simulink model "may9js"  (R2015a)
settings: Solver=ode4  StartTime=0.0  StopTime=inf  FixedStep=BKIN_STEP_TIME  RelTol=1e-3
StartFcn:
  |  warndlg('Dexterit-E models cannot run under simulation. Please compile your model and run it from within Dexterit-E.');set_param(bdroot,'SimulationCommand','stop')
model workspace (MAT data in the model file):
  BARRIER_ROW = 5
  BKIN_KINEMATIC_FRAME_SIZE = 400
  BKIN_STEP_TIME = 0.00025
  CIRCLE_ROW = 2
  CIRCLE_STROKE = 10
  CIRCLE_STROKE_W = 11
  E_BARRIER_HIT = 6
  E_COLLISION_HIT = 7
  E_ENTER_PRESHOT_AREA = 2
  E_ENTER_START_AREA = 12
  E_EXIT = 13
  E_EXIT_PRESHOT_AREA = 10
  E_GOAL_HIT = 8
  E_GOAL_REACHED = 5
  E_NO_EVENT = 0
  E_PRESHOT_ROW = 4
  E_TARGET_OUT_OF_BOUNDS = 9
  E_TRIAL_BEGIN = 1
  E_TRIAL_ENDED = 3
  FIRST_STATE_FILL = 9
  FORCE_MULTIPLIER = 1
  F_BUMP = 1
  GOAL_ROW = 8
  GOAL_TIME = 15
  HEIGHT = 6
  INVISIBLE_FILL = 15
  LOAD_ROW = 4
  MASS_BARRIER = 6
  MASS_CIRCLE = 2
  MASS_RECT = 3
  NEW_FLOAT = 10
  NEW_ROW = 9
  NEW_TEXTSIZE = 11
  PERT_DUR = 5
  PERT_RAMP = 4
  PRESHOT_ROW = 7
  RADIUS_LOG = 4
  RADIUS_VIS = 5
  RECT_FILL = 12
  RECT_ROW = 3
  RECT_STROKE = 13
  RECT_STROKE_W = 14
  ROTATION = 7
  SECONDS = 1
  SECOND_STATE_FILL = 8
  SHOT_READY_TIME = 13
  SHOT_SET_TIME = 14
  START_HOLD_TIME = 12
  START_ROW = 6
  TRIAL_FAILURE = 11
  WIDTH = 3
  col_x = 1
  col_y = 2
undefined symbols (not defined in the file): slselsubs
libraries: Video x7, General x3, KINARM_loads x2, KINARM_EP_loads x1, KINARM_general x1, simulink x1, slrtlib x1
(part 1 of 4)
settings Model: ModifiedComment=chris -- Wed Feb 16 09:18:30 2005 -- Version 1.1384  ModifiedHistory=Feb 16/05 - Add error repeat, add offset ramp  ExtModeArmWhenConnect=off  ExtModeLogAll=off  Creator=Chris Grebeldinger  LastModifiedBy=User
settings SolverCC: AutoInsertRateTranBlk=on
settings DataIOCC: LimitDataPoints=off  SignalLoggingSaveFormat=ModelDataLogs  SaveOutput=off  SaveTime=off  SignalLoggingName=sigsOut
settings OptimizationCC: BlockReduction=off  BooleanDataType=off  OptimizeBlockIOStorage=off  BufferReuse=off  GlobalBufferReuse=off  ExpressionFolding=off  ExpressionDepthLimit=2147483647  LocalBlockOutputs=off  InitFltsAndDblsToZero=on
settings DebuggingCC: SaveWithParameterizedLinksMsg=none  UnderspecifiedInitializationDetection=Classic  MergeDetectMultiDrivingBlocksExec=none  SignalResolutionControl=TryResolveAllWithWarning  MultiTaskDSMMsg=warning  FcnCallInpInsideContextMsg=EnableAllAsWarning  BusObjectLabelMismatch=none  StateNameClashWarn=warning  StrictBusMsg=ErrorOnBusTreatedAsVector
settings HardwareCC: ProdIntDivRoundTo=Zero  ProdEndianess=LittleEndian  ProdLongLongMode=on  ProdHWDeviceType=Generic->32-bit x86 compatible  TargetHWDeviceType=32-bit Generic
settings SFSimCC: SimParseCustomCode=off
settings RTWCC: Description=Simulink Real-Time  SystemTargetFile=slrt.tlc  TemplateMakefile=slrt_default_tmf  CodeExecutionProfiling=on  RTWCompilerOptimization=on
settings CodeAppCC: MaxIdLength=63
settings SimulinkRealTimeCC: TargetFcnLib=ansi_tfl_tmw.mat  GeneratePreprocessorConditionals=Disable all

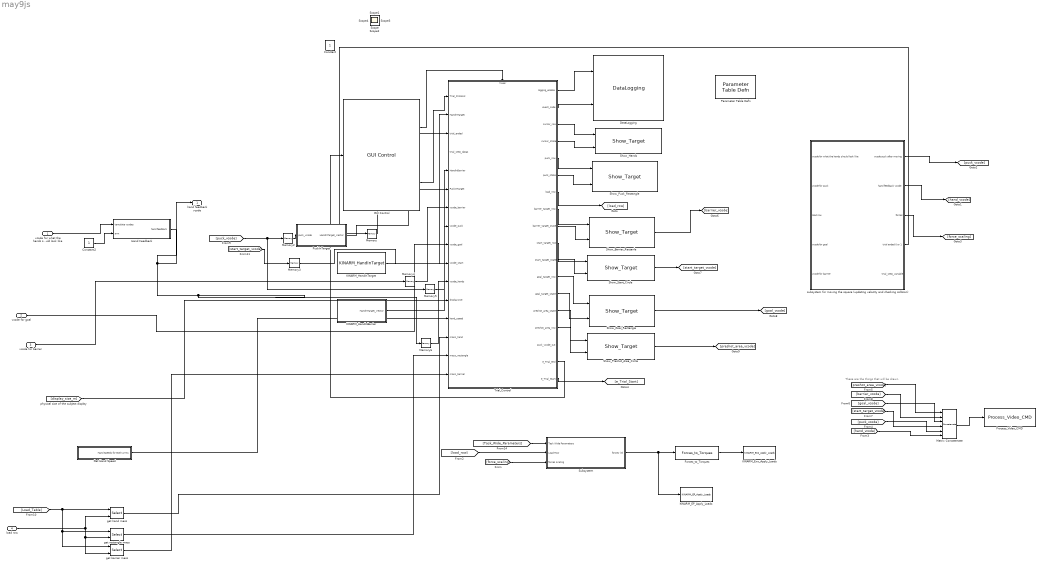
== system may9js ==
  note: These are the things that will be drawn
  vcode for what the hands should look like : Inport  PortDimensions=[1 70]
  vcode for goal : Inport  Port=2  PortDimensions=[1 70]
  vcode for barrier : Inport  Port=3  PortDimensions=[1 70]
  load row : Inport  Port=4
  Constant2 : Constant
  DataLogging : General/DataLogging  log_event_codes=on  log_analog_inputs=off  show_time_remaining=off  ecat_include=on
  Forces_to_Torques : KINARM_loads/Forces_to_Torques
  GUI Control : General/GUI Control  task_version=1.0  show_repeat_trial_flag=off  use_custom_tp=off  target_type_str=Circle  Target_Type=1  XYcols=[1 2]  Vcols=3  Lcols=4  indices_padding=[0 0 0 0;0 0 0 0]  target_table_rows=64  load_table_rows=20  tp_table_rows=100
  Get Hand Speed : Subsystem
  Hand Feedback : Subsystem
  KINARM_EP_Apply_Loads : KINARM_EP_loads/KINARM_EP_Apply_Loads  up_duration=1500  down_duration=1500  max_force=20
  KINARM_Exo_Apply_Loads : KINARM_loads/KINARM_Exo_Apply_Loads  up_duration=1500  down_duration=1500  max_torque=5  limit_motors=off
  KINARM_HandInBarrier : Subsystem  AncestorBlock=KINARM_general/KINARM_HandInTarget  mask(KINARM_HandInTarget){use_dominant_hand=on, target_type=Rectangle, num_states=1, attribcol1=[WIDTH HEIGHT ROTATION], attribcol2=[0 0 0], attribcol3=[0 0 0], attribcol4=[0 0 0], attribcol5=[0 0 0]}
      mask prompts: use_dominant_hand "Use "arm to be assessed"?"; target_type "Type of Target"; num_states "Number of Target States"; attribcol1 "State 1 Target Table Column(s)"; attribcol2 "State 2 Target Table Column(s)"; attribcol3 "State 3 Target Table Column(s)"; attribcol4 "State 4 Target Table Column(s)"; attribcol5 "State 5 Target Table Column(s)"
      mask help: This block returns a vector or array corresponding to the Target_Table rows indicating whether the specified hand is in (=1) or out (=0) of each of the targets.
      mask init:
      | block_path = gcb;  % store block path, as gcb may change with block operations
      | 
      | %%% Get the model's workspace, because it is required to evaluate constants from the Parameter Table Def'n block
      | modelName=bdroot(block_path);
      | modelWorkspace = get_param(modelName, 'ModelWorkspace');
      | 
      | %%% Handle background colours if link status changes.  
      | checkBackgroundColour(block_path, 'KINARM_general');
      | 
      | %%% create the names of the input and output ports to display on the mask
      | % Select only the desired states for output. The output port is also renamed to reflect 
      | % whether the output is a vector (in the case of a single state) or an array (of vectors, 
      | % one for each of multiple states).
      | 
      | numStates = str2double( get_param(block_path, 'num_states') );
      | 
      | if numStates == 1
      | 	set_param([block_path '/Selected States'], 'Value', '[1]');
      | 	outputname = 'HandInTarget_Vector';
      | elseif numStates == 2
      | 	set_param([block_path '/Selected States'], 'Value', '[1,2]');
      | 	outputname = 'HandInTarget_Array';
      | elseif numStates == 3
      | 	set_param([block_path '/Selected States'], 'Value', '[1,2,3]');
      | 	outputname = 'HandInTarget_Array';
      | elseif numStates == 4
      | 	set_param([block_path '/Selected States'], 'Value', '[1,2,3,4]');
      | 	outputname = 'HandInTarget_Array';
      | else
      | 	set_param([block_path '/Selected States'], 'Value', '[1,2,3,4,5]');
      | 	outputname = 'HandInTarget_Array';
      | end
      | output_block=char(find_system(gcb,'LookUnderMasks','all','FollowLinks','on','SearchDepth',1,'BlockType','Outport'));
      | set_param(output_block, 'Name', outputname);
      | 
      | 
      | %%%%%%%%%%%%%%%%%%%%%%%%%%%%%%%%%%%%%%%%%%%%%%%%%%%%%%%%%%%%%
      | %%% Check and format the input strings for the vectors of column entires
      | targetTypeStr=get_param(block_path, 'target_type');
      | 
      | switch targetTypeStr(1:3)
      | 	case 'Cir',		numCol = 1;
      | 	case 'Ell',		numCol = 3;
      |     case 'Rec',		numCol = 3;
      |     case 'Lin',		numCol = 3;
      |     case 'Tri',		numCol = 4;
      | 	otherwise,		numCol = 1;
      | end
      | 
      | for ii = 1:numStates
      | 	variableName = ['attribcol' num2str(ii)];
      | 	attribcoltext = get_param(block_path, variableName);
      | 	attribcoltext = checkUserInputVectorLength(attribcoltext, numCol);
      | 	set_param(block_path, variableName, attribcoltext);
      | end
      | 
      | for ii = 1+numStates:5
      | 	variableName = ['attribcol' num2str(ii)];
      |     if numCol == 1
      |         outstr = '[0]';
      |     else
      |         outstr = mat2str(zeros(1, numCol));
      |     end
      |     set_param(block_path, variableName, outstr);
      | end
      | 
      | %%%%%%%%%%%%%%%%%%%%%%%%%%%%%%%%%%%%%%%%%%%%%%%%%%%%%%%%%%%%%
      | %%% Create the text to show on the mask
      | numStates = str2num(get_param(block_path, 'num_states'));
      | columntext='(columns: ';
      | 
      | for ii = 1:numStates
      | 	variableName = ['attribcol' num2str(ii)];
      | 	attribcolString = get_param(block_path, variableName);
      | 	if isempty(modelWorkspace)
      | 		% if the block is part of a library, then modelWorkspace will be empty and the other code to evaluate attribcolStringEval will fail
      | 		attribcolStringEval = '3';
      | 	else
      | 		[attribcolValue, errorMessage] = BKINevalin(modelWorkspace, attribcolString);
      | 		attribcolStringEval = mat2str( attribcolValue );
      | 	end
      | 	if ii > 1
      | 		columntext = [columntext, '; ', attribcolStringEval];
      | 	else
      | 		columntext = [columntext, attribcolStringEval];
      | 	end
      | end
      | 
      | % Add formatting spaces so that the mask looks nice
      | columntext=strvcat([columntext ')'],' ', ' ');
      mask Help:
      | Used to determine if the hand (fingertip) is in any of the targets in the Target_Table.
      | <P>
      | <B><I>Use of this block requires that the DataLogging block (General library) be set to log KINARM data.</I></B>
      | 
      | <H2>Library </H2>
      | KINARM general
      | 
      | <H2>Description </H2>
      | This block returns a vector or array corresponding to the Target_Table rows indicating whether the specified hand (i.e. fingertip) is in or out of each of the targets.  Each element in the output vector or output array will be either a 0 (hand not in target) or a 1 (hand in target).
      | <P>
      | A vector is returned if only one target state is specified in each target row (see Parameters and Dialog Box), with each index of the vector corresponding to a row in the target table.  An array is returned if more than one target state is specified in a target row, with each row of the array corresponding to a target row and each column corresponding to the nth target state specified in each target row.
      | <P>
      | The output vector or array is typically used by a stateflow chart to affect behavior of the system.  Because this block returns hand-in-target information for all targets in the target table, multiple targets can be monitored at once (i.e. the Stateflow chart could have certain transitions that occur if the hand is in one target and other transitions if it is in a different target).  Likewise, because this block returns hand-in-target information for multiple states of a single target, those multiple states can be monitored simultaneously.
      | <P>
      | Because the KINARM_HandInTarget block returns information for only one hand, two copies of this block are required if information for both hands is desired.
      | <P>
      | 
      | <H2>Parameters and Dialog Box</H2>
      | <B>Use "arm to be assessed"?:</B> this checkbox determines which hand is used by this block. In Dexterit-E the operator selects the "arm to be assessed" using radio buttons.
      | When this box is checked the output of this block is derived from the hand information corresponding to the arm selection made by the operator in Dexterit-E.
      | When this box is unchecked the output of this block is derived from the contralateral arm.
      | (Note: to obtain information about both hands, then 2 separate copies of this block are required - one for each hand.)
      | <P>
      | <B>Type of Target:</B> Enter the type of target specified in the target table:
      | <P>
      | <B>Number of Target States:</B> Enter the number of target states specified in each target row.  Up to four target states are allowed per target row.
      | <P>
      | <B>State <n> Target Table Columns:</B> Enter the columns in the Target Table that specify the relevant target attributes.  Do this for each target state.
      | For a circle, enter the columns corresponding to logical radius (e.g. 4)
      | <BR>For an ellipse, enter the columns corresponding to major radius, minor radius, rotation angle (e.g. [4, 5, 6]).
      | <BR>For a rectangle, enter the columns corresponding to length, height, and rotation angle (e.g. [4, 5, 6]).
      | <BR>For a line, enter the columns corresponding to stroke width, endpoint in x, and endpoint in y (e.g. [3, 4, 5]).
      | <BR>For a triangle, enter the columns corresponding to length, height, peak offset, and rotation angle (e.g. [4, 5, 6, 7]).
      | 
      | <H2>Examples</H2>
      | <B>Example 1.</B>  Suppose a target row will be used to define 1 state for a circle type target and the radius of the visual target is the same radius to be used for determination of hand-in-target.  The related Target Table column is: column 6 = radius.  For this example, "State 1 Target Table Columns" would equal [6].
      | <P>
      | 
      | <B>Example 2.</B>  Suppose a target row will be used to define 1 state for a circle type target, but the radius of the visual target will be different than the radius to be used for determination of hand-in-target.  This option allows independent control over the size of the visual target versus the accuracy needed to be considered "in the target".  The related Target Table columns are: column 6 = radius1 (i.e. radius to target to be drawn); column 7 = radius2 (i.e. radius to be used for hand-in-target) .  For this example, "State 1 Target Table Columns" would equal [7].
      | <P>
      | <B>Example 3.</B>  Suppose a target row will be used to define 2 states for a circle type target, where the radius of the visual target will be a constant, but depending on the state of the system, one of 2 other and different radii will be used for determination of hand-in-target.  The related Target Table columns are: column 6 = radius1 (i.e. radius to target to be drawn); column 7 = radius2 (i.e. radius to be used for hand-in-target for state 1); column 8 = radius3 (i.e. radius to be used for hand-in-target for state 2).  For this example, "State 1 Target Table Columns" would equal [7], while "State 2 Target Table Columns" would equal [8].
      | <P>
      | 
      | <H2>Related Blocks </H2>
      | DataLogging
      mask TypeOptions target_type: Circle | Ellipse | Rectangle | Line | Triangle
      mask Callback target_type:
      | %%%%
      | % Because of bugs iN R2007, R2010a and R2013a (which have been reported to Mathworks), the following code
      | % is required here because in the Initialization Section it will ONLY correctly update those Mask Parameters that are hidden
      | % when the OK button is clicked (NOTE: the initialization code will correctly update all Mask Parameters when the Apply button
      | % is clicked, the bug is that it should also update everything when the OK button is clicked in the absence of an Apply click)
      | %
      | % Adding a set_param call which updates one of the mask parameters will call the initialization code to run, which "avoids"
      | % this bug. This code should be removed once Mathworks has fixed this bug.
      | 
      | temp = get_param(gcb, 'target_type');
      | set_param(gcb, 'target_type', temp);
      mask TypeOptions num_states: 1 | 2 | 3 | 4 | 5
      mask Callback num_states:
      | num_states = str2num(get_param(gcb, 'num_states'));
      | vis = get_param(gcb, 'MaskVisibilities');
      | 
      | % Select only the desired states for output. The output port is also renamed to reflect
      | % whether the output is a vector (in the case of a single state) or an array (of vectors,
      | % one for each of multiple states).
      | output_block=char(find_system(gcb, 'LookUnderMasks', 'all', 'FollowLinks', 'on', 'SearchDepth', 1, 'BlockType', 'Outport'));
      | 
      | if num_states == 1
      | % % % 	set_param([gcb '/Selected States'], 'Value', '[1]');
      | % % % 	set_param(output_block, 'Name', 'HandInTarget_Vector');
      | 	vis{5} = 'off';
      | 	vis{6} = 'off';
      | 	vis{7} = 'off';
      | 	vis{8} = 'off';
      | elseif num_states == 2
      | % % % 	set_param([gcb '/Selected States'], 'Value', '[1,2]');
      | % % % 	set_param(output_block, 'Name', 'HandInTarget_Array');
      | 	vis{5} = 'on';
      | 	vis{6} = 'off';
      | 	vis{7} = 'off';
      | 	vis{8} = 'off';
      | elseif num_states == 3
      | % % % 	set_param([gcb '/Selected States'], 'Value', '[1,2,3]');
      | % % % 	set_param(output_block, 'Name','HandInTarget_Array');
      | 	vis{5} = 'on';
      | 	vis{6} = 'on';
      | 	vis{7} = 'off';
      | 	vis{8} = 'off';
      | elseif num_states == 4
      | % % % 	set_param([gcb '/Selected States'], 'Value', '[1,2,3,4]');
      | % % % 	set_param(output_block, 'Name','HandInTarget_Array');
      | 	vis{5} = 'on';
      | 	vis{6} = 'on';
      | 	vis{7} = 'on';
      | 	vis{8} = 'off';
      | else
      | % % % 	set_param([gcb '/Selected States'], 'Value', '[1,2,3,4,5]');
      | % % % 	set_param(output_block, 'Name', 'HandInTarget_Array');
      | 	vis{5} = 'on';
      | 	vis{6} = 'on';
      | 	vis{7} = 'on';
      | 	vis{8} = 'on';
      | end
      | set_param(gcb, 'MaskVisibilities', vis);
      mask Display:
      | disp(columntext);
      | port_label('output',1,outputname);
  KINARM_HandInTarget : KINARM_general/KINARM_HandInTarget  use_dominant_hand=on  target_type=Circle  num_states=1  attribcol1=[RADIUS_LOG]  attribcol2=[0]  attribcol3=[0]  attribcol4=[0]  attribcol5=[0]
  Matrix Concatenate : Concatenate  NumInputs=6  Mode=Multidimensional array
  Memory{,2..6} (6 alike) : Memory
  Parameter Table Defn : General/Parameter Table Defn  ShowInLibBrowser=0
  Process_Video_CMD : Video/Process_Video_CMD  video_delay=0
  PuckInTarget : Subsystem  AncestorBlock=KINARM_general/KINARM_HandInTarget  mask(KINARM_HandInTarget){use_dominant_hand=on, target_type=Rectangle, num_states=1, attribcol1=[WIDTH HEIGHT ROTATION], attribcol2=[0 0 0], attribcol3=[0 0 0], attribcol4=[0 0 0], attribcol5=[0 0 0]}
      mask prompts: use_dominant_hand "Use "arm to be assessed"?"; target_type "Type of Target"; num_states "Number of Target States"; attribcol1 "State 1 Target Table Column(s)"; attribcol2 "State 2 Target Table Column(s)"; attribcol3 "State 3 Target Table Column(s)"; attribcol4 "State 4 Target Table Column(s)"; attribcol5 "State 5 Target Table Column(s)"
      mask help: This block returns a vector or array corresponding to the Target_Table rows indicating whether the specified hand is in (=1) or out (=0) of each of the targets.
      mask init: same as may9js/KINARM_HandInBarrier
      mask Help:
      | Used to determine if the hand (fingertip) is in any of the targets in the Target_Table.
      | <P>
      | <B><I>Use of this block requires that the DataLogging block (General library) be set to log KINARM data.</I></B>
      | 
      | <H2>Library </H2>
      | KINARM general
      | 
      | <H2>Description </H2>
      | This block returns a vector or array corresponding to the Target_Table rows indicating whether the specified hand (i.e. fingertip) is in or out of each of the targets.  Each element in the output vector or output array will be either a 0 (hand not in target) or a 1 (hand in target).
      | <P>
      | A vector is returned if only one target state is specified in each target row (see Parameters and Dialog Box), with each index of the vector corresponding to a row in the target table.  An array is returned if more than one target state is specified in a target row, with each row of the array corresponding to a target row and each column corresponding to the nth target state specified in each target row.
      | <P>
      | The output vector or array is typically used by a stateflow chart to affect behavior of the system.  Because this block returns hand-in-target information for all targets in the target table, multiple targets can be monitored at once (i.e. the Stateflow chart could have certain transitions that occur if the hand is in one target and other transitions if it is in a different target).  Likewise, because this block returns hand-in-target information for multiple states of a single target, those multiple states can be monitored simultaneously.
      | <P>
      | Because the KINARM_HandInTarget block returns information for only one hand, two copies of this block are required if information for both hands is desired.
      | <P>
      | 
      | <H2>Parameters and Dialog Box</H2>
      | <B>Use "arm to be assessed"?:</B> this checkbox determines which hand is used by this block. In Dexterit-E the operator selects the "arm to be assessed" using radio buttons.
      | When this box is checked the output of this block is derived from the hand information corresponding to the arm selection made by the operator in Dexterit-E.
      | When this box is unchecked the output of this block is derived from the contralateral arm.
      | (Note: to obtain information about both hands, then 2 separate copies of this block are required - one for each hand.)
      | <P>
      | <B>Type of Target:</B> Enter the type of target specified in the target table:
      | <P>
      | <B>Number of Target States:</B> Enter the number of target states specified in each target row.  Up to four target states are allowed per target row.
      | <P>
      | <B>State <n> Target Table Columns:</B> Enter the columns in the Target Table that specify the relevant target attributes.  Do this for each target state.
      | For a circle, enter the columns corresponding to logical radius (e.g. 4)
      | <BR>For an ellipse, enter the columns corresponding to major radius, minor radius, rotation angle (e.g. [4, 5, 6]).
      | <BR>For a rectangle, enter the columns corresponding to length, height, and rotation angle (e.g. [4, 5, 6]).
      | <BR>For a line, enter the columns corresponding to stroke width, endpoint in x, and endpoint in y (e.g. [3, 4, 5]).
      | <BR>For a triangle, enter the columns corresponding to length, height, peak offset, and rotation angle (e.g. [4, 5, 6, 7]).
      | 
      | <H2>Examples</H2>
      | <B>Example 1.</B>  Suppose a target row will be used to define 1 state for a circle type target and the radius of the visual target is the same radius to be used for determination of hand-in-target.  The related Target Table column is: column 6 = radius.  For this example, "State 1 Target Table Columns" would equal [6].
      | <P>
      | 
      | <B>Example 2.</B>  Suppose a target row will be used to define 1 state for a circle type target, but the radius of the visual target will be different than the radius to be used for determination of hand-in-target.  This option allows independent control over the size of the visual target versus the accuracy needed to be considered "in the target".  The related Target Table columns are: column 6 = radius1 (i.e. radius to target to be drawn); column 7 = radius2 (i.e. radius to be used for hand-in-target) .  For this example, "State 1 Target Table Columns" would equal [7].
      | <P>
      | <B>Example 3.</B>  Suppose a target row will be used to define 2 states for a circle type target, where the radius of the visual target will be a constant, but depending on the state of the system, one of 2 other and different radii will be used for determination of hand-in-target.  The related Target Table columns are: column 6 = radius1 (i.e. radius to target to be drawn); column 7 = radius2 (i.e. radius to be used for hand-in-target for state 1); column 8 = radius3 (i.e. radius to be used for hand-in-target for state 2).  For this example, "State 1 Target Table Columns" would equal [7], while "State 2 Target Table Columns" would equal [8].
      | <P>
      | 
      | <H2>Related Blocks </H2>
      | DataLogging
      mask TypeOptions target_type: Circle | Ellipse | Rectangle | Line | Triangle
      mask Callback target_type:
      | %%%%
      | % Because of bugs iN R2007, R2010a and R2013a (which have been reported to Mathworks), the following code
      | % is required here because in the Initialization Section it will ONLY correctly update those Mask Parameters that are hidden
      | % when the OK button is clicked (NOTE: the initialization code will correctly update all Mask Parameters when the Apply button
      | % is clicked, the bug is that it should also update everything when the OK button is clicked in the absence of an Apply click)
      | %
      | % Adding a set_param call which updates one of the mask parameters will call the initialization code to run, which "avoids"
      | % this bug. This code should be removed once Mathworks has fixed this bug.
      | 
      | temp = get_param(gcb, 'target_type');
      | set_param(gcb, 'target_type', temp);
      mask TypeOptions num_states: 1 | 2 | 3 | 4 | 5
      mask Callback num_states:
      | num_states = str2num(get_param(gcb, 'num_states'));
      | vis = get_param(gcb, 'MaskVisibilities');
      | 
      | % Select only the desired states for output. The output port is also renamed to reflect
      | % whether the output is a vector (in the case of a single state) or an array (of vectors,
      | % one for each of multiple states).
      | output_block=char(find_system(gcb, 'LookUnderMasks', 'all', 'FollowLinks', 'on', 'SearchDepth', 1, 'BlockType', 'Outport'));
      | 
      | if num_states == 1
      | % % % 	set_param([gcb '/Selected States'], 'Value', '[1]');
      | % % % 	set_param(output_block, 'Name', 'HandInTarget_Vector');
      | 	vis{5} = 'off';
      | 	vis{6} = 'off';
      | 	vis{7} = 'off';
      | 	vis{8} = 'off';
      | elseif num_states == 2
      | % % % 	set_param([gcb '/Selected States'], 'Value', '[1,2]');
      | % % % 	set_param(output_block, 'Name', 'HandInTarget_Array');
      | 	vis{5} = 'on';
      | 	vis{6} = 'off';
      | 	vis{7} = 'off';
      | 	vis{8} = 'off';
      | elseif num_states == 3
      | % % % 	set_param([gcb '/Selected States'], 'Value', '[1,2,3]');
      | % % % 	set_param(output_block, 'Name','HandInTarget_Array');
      | 	vis{5} = 'on';
      | 	vis{6} = 'on';
      | 	vis{7} = 'off';
      | 	vis{8} = 'off';
      | elseif num_states == 4
      | % % % 	set_param([gcb '/Selected States'], 'Value', '[1,2,3,4]');
      | % % % 	set_param(output_block, 'Name','HandInTarget_Array');
      | 	vis{5} = 'on';
      | 	vis{6} = 'on';
      | 	vis{7} = 'on';
      | 	vis{8} = 'off';
      | else
      | % % % 	set_param([gcb '/Selected States'], 'Value', '[1,2,3,4,5]');
      | % % % 	set_param(output_block, 'Name', 'HandInTarget_Array');
      | 	vis{5} = 'on';
      | 	vis{6} = 'on';
      | 	vis{7} = 'on';
      | 	vis{8} = 'on';
      | end
      | set_param(gcb, 'MaskVisibilities', vis);
      mask Display:
      | disp(columntext);
      | port_label('output',1,outputname);
  Show_Barrier_Rectanle : Video/Show_Target  target_type=Rectangle  num_states=2  attribcol1=[FIRST_STATE_FILL RECT_STROKE RECT_STROKE_W WIDTH HEIGHT ROTATION]  attribcol2=[SECOND_STATE_FILL RECT_STROKE RECT_STROKE_W WIDTH HEIGHT ROTATION]  attribcol3=[0 0 0 0 0 0]  attribcol4=[0 0 0 0 0 0]  attribcol5=[0 0 0 0 0 0]  stateindices_padding=[0 0 0 0 0;0 0 0 0 0;0 0 0 0 0;0 0 0 0 0;0 0 0 0 0]  source=dialog  opacity=100  target_display=Both subject and operator displays  num_col=6
  Show_Goal_Rectangle : Video/Show_Target  target_type=Rectangle  num_states=3  attribcol1=[INVISIBLE_FILL RECT_STROKE RECT_STROKE_W WIDTH HEIGHT ROTATION]  attribcol2=[FIRST_STATE_FILL RECT_STROKE RECT_STROKE_W WIDTH HEIGHT ROTATION]  attribcol3=[SECOND_STATE_FILL RECT_STROKE RECT_STROKE_W WIDTH HEIGHT ROTATION]  attribcol4=[0 0 0 0 0 0]  attribcol5=[0 0 0 0 0 0]  stateindices_padding=[0 0 0 0 0;0 0 0 0 0;0 0 0 0 0;0 0 0 0 0;0 0 0 0 0]  source=dialog  opacity=100  target_display=Both subject and operator displays  num_col=6
  Show_Hands : Video/Show_Target  target_type=Circle  num_states=2  attribcol1=[FIRST_STATE_FILL CIRCLE_STROKE CIRCLE_STROKE_W WIDTH]  attribcol2=[SECOND_STATE_FILL CIRCLE_STROKE CIRCLE_STROKE_W WIDTH]  attribcol3=[0 0 0 0]  attribcol4=[0 0 0 0]  attribcol5=[0 0 0 0]  stateindices_padding=[0 0 0 0 0 0 0;0 0 0 0 0 0 0;0 0 0 0 0 0 0;0 0 0 0 0 0 0;0 0 0 0 0 0 0]  source=dialog  opacity=100  target_display=Both subject and operator displays  num_col=4
  Show_Preshot_Area_Circle : Video/Show_Target  target_type=Circle  num_states=3  attribcol1=[INVISIBLE_FILL CIRCLE_STROKE CIRCLE_STROKE_W WIDTH]  attribcol2=[FIRST_STATE_FILL CIRCLE_STROKE CIRCLE_STROKE_W WIDTH]  attribcol3=[SECOND_STATE_FILL CIRCLE_STROKE CIRCLE_STROKE_W WIDTH]  attribcol4=[0 0 0 0]  attribcol5=[0 0 0 0]  stateindices_padding=[0 0 0 0 0 0 0;0 0 0 0 0 0 0;0 0 0 0 0 0 0;0 0 0 0 0 0 0;0 0 0 0 0 0 0]  source=dialog  opacity=100  target_display=Both subject and operator displays  num_col=4
  Show_Puck_Rectangle : Video/Show_Target  target_type=Rectangle  num_states=3  attribcol1=[INVISIBLE_FILL RECT_STROKE RECT_STROKE_W WIDTH HEIGHT ROTATION]  attribcol2=[FIRST_STATE_FILL RECT_STROKE RECT_STROKE_W WIDTH HEIGHT ROTATION]  attribcol3=[SECOND_STATE_FILL RECT_STROKE RECT_STROKE_W WIDTH HEIGHT ROTATION]  attribcol4=[0 0 0 0 0 0]  attribcol5=[0 0 0 0 0 0]  stateindices_padding=[0 0 0 0 0;0 0 0 0 0;0 0 0 0 0;0 0 0 0 0;0 0 0 0 0]  source=dialog  opacity=100  target_display=Both subject and operator displays  num_col=6
  Show_Start_Circle : Video/Show_Target  target_type=Circle  num_states=3  attribcol1=[INVISIBLE_FILL CIRCLE_STROKE CIRCLE_STROKE_W WIDTH]  attribcol2=[FIRST_STATE_FILL CIRCLE_STROKE CIRCLE_STROKE_W WIDTH]  attribcol3=[SECOND_STATE_FILL CIRCLE_STROKE CIRCLE_STROKE_W WIDTH]  attribcol4=[0 0 0 0]  attribcol5=[0 0 0 0]  stateindices_padding=[0 0 0 0 0 0 0;0 0 0 0 0 0 0;0 0 0 0 0 0 0;0 0 0 0 0 0 0;0 0 0 0 0 0 0]  source=dialog  opacity=100  target_display=Both subject and operator displays  num_col=4
  Subsystem : Subsystem
  Trial_Control : Stateflow chart  TreatAsAtomicUnit=on
      settings: PermitHierarchicalResolution=ParametersOnly
  get barrier mass : Selector  NumberOfDimensions=2  IndexOptions=Index vector (port),Index vector (dialog)  Indices=MASS_RECT,MASS_RECT  OutputSizes=1,1
  get hand mass : Selector  NumberOfDimensions=2  IndexOptions=Index vector (port),Index vector (dialog)  Indices=MASS_CIRCLE,MASS_CIRCLE  OutputSizes=1,1
  get rectangle mass : Selector  NumberOfDimensions=2  IndexOptions=Index vector (port),Index vector (dialog)  Indices=MASS_RECT,MASS_RECT  OutputSizes=1,1
  subsystem for moving the square (updating velocity and checking collision) : Subsystem
  hand feedback vcode : Outport
  Constant : Constant  IOType=siggen
  Scope{,1..4} (5 alike) : Scope
      Scope settings: TimeRange=auto  MaxDataPoints=5000  SaveToWorkspace=off  SaveName=ScopeData  YMin=-10.00000  YMax=10.00000  SampleTime=-1
      Scope1 settings: TimeRange=auto  MaxDataPoints=5000  SaveToWorkspace=off  YMin=-10.00000  YMax=10.00000  SampleTime=-1
      Scope2 settings: TimeRange=auto  MaxDataPoints=5000  SaveToWorkspace=off  SaveName=ScopeData2  YMin=-10.00000  YMax=10.00000  SampleTime=-1
      Scope3 settings: TimeRange=auto  MaxDataPoints=5000  SaveToWorkspace=off  SaveName=ScopeData3  YMin=-10.00000  YMax=10.00000  SampleTime=-1
      Scope4 settings: TimeRange=auto  MaxDataPoints=5000  SaveToWorkspace=off  SaveName=ScopeData4  YMin=-10.00000  YMax=10.00000  SampleTime=-1
  wires:
  Trial_Control/3(cursor_row) -> Show_Hands/1
  Trial_Control/5(puck_row) -> Show_Puck_Rectangle/1
  Trial_Control/6(puck_state) -> Show_Puck_Rectangle/2
  Forces_to_Torques/1 -> KINARM_Exo_Apply_Loads/1
  Trial_Control/1(logging_enable) -> DataLogging/1
  Trial_Control/7(load_row) -> [load_row]
  Trial_Control/17(e_Trial_End) -> GUI Control/1
  Trial_Control/4(cursor_state) -> Show_Hands/2
  GUI Control/1 -> Trial_Control/Trigger
  Matrix Concatenate/1 -> Process_Video_CMD/1
  subsystem for moving the square (updating velocity and checking collision)/1(vcode puck after moving) -> [puck_vcode]
  subsystem for moving the square (updating velocity and checking collision)/3(forces) -> [force_scaling]
  subsystem for moving the square (updating velocity and checking collision)/2(hand feedback vcode) -> [hand_vcode]
  Trial_Control/2(event_code) -> DataLogging/2
  Subsystem/1(forces (N)) -> KINARM_EP_Apply_Loads/1, Forces_to_Torques/1
  [Task_Wide_Parameters] -> Subsystem/1(Task Wide Parameters)
  [load_row] -> Subsystem/2(Load Row)
  [force_scaling] -> Subsystem/3(forces scaling)
  Trial_Control/8(barrier_target_row) -> Show_Barrier_Rectanle/1
  Trial_Control/9(barrier_target_state) -> Show_Barrier_Rectanle/2
  Trial_Control/10(start_target_row) -> Show_Start_Circle/1
  Trial_Control/11(start_target_state) -> Show_Start_Circle/2
  Trial_Control/12(goal_target_row) -> Show_Goal_Rectangle/1
  Trial_Control/13(goal_target_state) -> Show_Goal_Rectangle/2
  KINARM_HandInTarget/1 -> Trial_Control/2(HandInTarget)
  GUI Control/2 -> Trial_Control/1(Trial_Protocol)
  subsystem for moving the square (updating velocity and checking collision)/4(trial ended 0 or 1) -> Memory/1
  Memory/1 -> Trial_Control/3(trial_ended)
  Show_Barrier_Rectanle/1 -> [barrier_vcode]
  Show_Start_Circle/1 -> [start_target_vcode]
  Trial_Control/14(preshot_area_state) -> Show_Preshot_Area_Circle/2
  Trial_Control/15(preshot_area_row) -> Show_Preshot_Area_Circle/1
  [hand_vcode] -> Matrix Concatenate/6
  [puck_vcode] -> Matrix Concatenate/5
  [preshot_area_vcode] -> Matrix Concatenate/1
  [barrier_vcode] -> Matrix Concatenate/2
  [goal_vcode] -> Matrix Concatenate/3
  [start_target_vcode] -> Matrix Concatenate/4
  KINARM_HandInBarrier/1(HandInTarget_Vector) -> Trial_Control/5(HandInBarrier)
  [puck_vcode] -> Memory5/1, Memory2/1
  PuckInTarget/1(HandInTarget_Vector) -> Trial_Control/6(PuckInTarget)
  Memory2/1 -> PuckInTarget/1(puck_vcode)
  Trial_Control/18(e_Trial_Start) -> [e_Trial_Start]
  Constant2/1 -> Hand Feedback/2(arm)
  vcode for what the hands should look like/1 -> Hand Feedback/1(template vcodes)
  Hand Feedback/1(hand feedback) -> Memory6/1, hand feedback vcode/1
  vcode for goal/1 -> Trial_Control/9(vcode_goal)
  vcode for barrier/1 -> Memory4/1
  Get Hand Speed/1(Hand Speeds for Both Arms) -> Trial_Control/13(hand_speed)
  [Load_Table] -> get barrier mass/1, get rectangle mass/1, get hand mass/1
  get rectangle mass/1 -> Trial_Control/15(mass_rectangle)
  get barrier mass/1 -> Trial_Control/16(mass_barrier)
  load row/1 -> get barrier mass/2, get rectangle mass/2, get hand mass/2
  get hand mass/1 -> Trial_Control/14(mass_hand)
  [display_size_m] -> Trial_Control/12(displaysize)
  Memory5/1 -> Trial_Control/8(vcode_puck)
  Memory4/1 -> Trial_Control/7(vcode_barrier)
  Memory6/1 -> Trial_Control/11(vcode_hands)
  Show_Goal_Rectangle/1 -> [goal_vcode]
  Show_Preshot_Area_Circle/1 -> [preshot_area_vcode]
  [start_target_vcode] -> Memory3/1
  Memory3/1 -> Trial_Control/10(vcode_start)

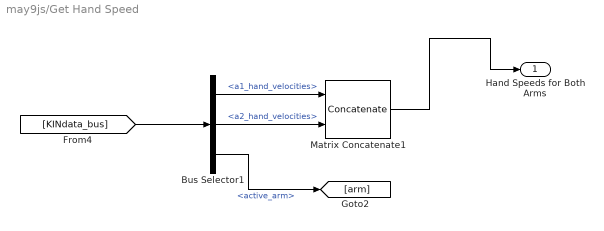
== system may9js/Get Hand Speed ==
  Bus Selector1 : BusSelector  OutputSignals=Robot1.a1_hand_velocities,Robot2.a2_hand_velocities,KINDataGeneral.active_arm
  Matrix Concatenate1 : Concatenate  Mode=Multidimensional array
  Hand Speeds for Both Arms : Outport
  wires:
  [KINdata_bus] -> Bus Selector1/1
  Bus Selector1/1 -> Matrix Concatenate1/1  "<a1_hand_velocities>"
  Matrix Concatenate1/1 -> Hand Speeds for Both Arms/1
  Bus Selector1/2 -> Matrix Concatenate1/2  "<a2_hand_velocities>"
  Bus Selector1/3 -> [arm]  "<active_arm>"

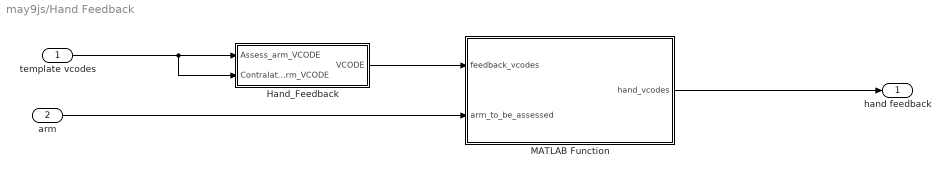
== system may9js/Hand Feedback ==
  template vcodes : Inport
  arm : Inport  Port=2
  Hand_Feedback : Subsystem  AncestorBlock=KINARM_general/Hand_Feedback  mask(Hand_Feedback){feedback_cntl_src=style and status}
      mask prompts: feedback_cntl_src "Task Program control of style and status"
      mask help:
      | This block controls various options for hand feedback (i.e. fingertip position)  to be shown to the subject.
      |
      | Task Program control of style and status refers to whether the Program Task will explicity control the style and/or status of the hand feedback.
      mask init:
      | block_path = gcb;  % store block path, as gcb may change with block operations
      | 
      | %%% Handle background colours if link status changes.  
      | checkBackgroundColour(block_path, 'KINARM_general');
      | 
      | 
      | feedback_cntl_source=get_param(gcb,'feedback_cntl_src');
      | 
      | if feedback_cntl_source(1:4)=='none'
      |     block1type='Constant';
      |     block2type='Constant';
      |     block3type='Constant';
      | elseif feedback_cntl_source(1:4)=='stat'
      |     block1type='Constant';
      |     block2type='Constant';
      |     block3type='Inport';
      | else 
      |     block1type='Inport';
      |     block2type='Inport';
      |     block3type='Constant';
      | end
      | 
      | hasOldName1 = ~isempty(find_system(gcb, 'FollowLinks', 'on', 'LookUnderMasks', 'all', 'name', 'Dom_VCODE'));
      | hasOldName2 = ~isempty(find_system(gcb, 'FollowLinks', 'on', 'LookUnderMasks', 'all', 'name', 'non-Dom_VCODE'));
      | 
      | block1name='Assess_arm_VCODE';
      | block2name='Contralateral_arm_VCODE';
      | block1path=[gcb '/' block1name];
      | block2path=[gcb '/' block2name];
      | 
      | if hasOldName1
      | 	set_param([gcb '/Dom_VCODE'],'name', block1name);
      | end
      | 
      | if hasOldName2
      | 	set_param([gcb '/non-Dom_VCODE'],'name', block2name);
      | end
      | 
      | if ~strcmp(get_param(block1path,'blocktype'),block1type)
      | 	pos=get_param(block1path,'position');
      | 	delete_line(gcb, [block1name '/1'], 'Reshape/1');
      | 	delete_block(block1path);
      | 	add_block(['built-in/' block1type], block1path,'Name',block1name);
      | 	set_param(block1path,'position',pos);
      | 	add_line(gcb, [block1name '/1'], 'Reshape/1');
      | end
      | 
      | if ~strcmp(get_param(block2path,'blocktype'),block2type)
      | 	pos=get_param(block2path,'position');
      | 	delete_line(gcb, [block2name '/1'], 'Reshape1/1');
      | 	delete_block(block2path);
      | 	add_block(['built-in/' block2type],block2path,'Name',block2name);
      | 	set_param(block2path,'position',pos);
      | 	add_line(gcb, [block2name '/1'], 'Reshape1/1');
      | end
      | 
      | block3name='feedback_status';
      | block3path=[gcb '/' block3name];
      | if ~strcmp(get_param(block3path,'blocktype'),block3type)
      | 	pos=get_param(block3path,'position');
      | 	delete_line(gcb, [block3name '/1'], 'FeedFwdArm/3');
      | 	delete_block(block3path);
      | 	add_block(['built-in/' block3type],block3path,'Name',block3name);
      | 	set_param(block3path,'position',pos);
      | 	add_line(gcb, [block3name '/1'], 'FeedFwdArm/3');
      | end
      | 
      | if feedback_cntl_source(1:4)=='none'
      | 	set_param(block1path,'Value','[1:70]');
      | 	set_param(block2path,'Value','[71:140]');
      | elseif feedback_cntl_source(1:4)=='stat'
      | 	set_param(block1path,'Value','[1:70]');
      | 	set_param(block2path,'Value','[71:140]');
      | end
      mask Help:
      | Creates VCODE for drawing hand position (fingertip).
      | <P>
      | <H2>Library </H2>
      | KINARM general
      | 
      | <H2>Description </H2>
      | This block controls various options for drawing hand feedback.  (Note: although it is called hand feedback, it is actually the fingertip position that is shown).  Three options are available (as chosen in the Parameters and Dialog box):
      | <P>
      | (i) GUI control of feedback style and status
      | <Blockquote>
      | No inputs are required for this option.  The Task Program has no control over the style or status of the hand feedback.
      | </Blockquote>
      | (ii) Task Program control of feedback status and GUI control of style
      | <Blockquote>
      | If Task Program control of feedback status is chosen, then one input appears for this block:<P>
      | <B> feedback_status: </B> this scalar input dynamically controls the status of the hand feedback as per the following:
      | <P>
      | 0 = (no hand feedback)<BR>
      | 1 = ("arm to be assessed" hand feedback only)<BR>
      | 2 = (contralateral arm hand feedback only)<BR>
      | 3 = (hand feedback on for both hands)<BR>
      | </Blockquote>
      | (iii) Task Program control of both feedback style and status.
      | <Blockquote>
      | 
      | If Task Program control of feedback status and style is chosen, then two inputs appear for this block:<P>
      | <B> Assess_arm_VCODE: </B>  this vector input dynamically controls the status and style of the hand feedback for the "arm to be assessed" the operator selected in Dexterit-E.
      | <P>
      | <B> Contralateral_arm_VCODE:</B>  this vector input dynamically controls the status and style of the hand feedback for the contralateral hand.
      | <P>
      | For both the Assess_arm_VCODE and the Contralateral_arm_VCODE, the input vectors must be in the appropriate VCODE format (for more information on the details of a VCODE, please right click on the Show_Target block in the video library, "Look Under Mask" and open the Embedded Matlab function).  Note that the position information in the Dom_VCODE and non-Dom_VCODE are overwritten in this block, but all other aspects of the VCODE are passed through to the output.
      | </Blockquote>
      | Note that if Task Program control is chosen for either hand feedback status or style, the GUI will still override these settings if the Task Protocol specifies that it should do so.
      | <P>
      | There is one output from this block:
      | <P>
      | <B> VCODE: </B> this output is 2-row matrix containing 2 VCODEs.  The first VCODE is for the dominant hand feedback and the second VCODE is for the non-dominant hand feedback.  This output must go to the Process_Video_CMD block of the video library for the hand feedback to actually be shown (if any other visual targets are to be displayed, then this VCODE output must be concatenated with the other VCODES prior to connection to the Process_Video_CMD block - see Help for the Process_Video_CMD block for more information).
      | <H2>Parameters and Dialog Box</H2>
      | <B>Task Program control of style and status</B> refers to whether the Program Task will explicity control the style and/or status of the hand feedback.  The three options are: none, status only, or status and style.
      | <P>
      |  - Choosing none means that style and status are always controlled by the GUI.
      | <P>
      |  - Choosing status only means that the GUI always controls the hand feedback style, but also will create an input to this block allowing the end user to control the status dynamically.  Allowable input values are: 0 (no hand feedback), 1 (dominant hand feedback only), 2 (non-dominant hand feedback only) or 3 (hand feedback on for both hands)
      |  <P>
      | - Choosing status and style means that both the hand feedback status and style can be controlled dynamically by the Task Program.  If this option is selected, then two inputs will be created for this block: dominant VCODE and non-dominant VCODE.  These two inputs require a proper VCODE (e.g. from a Show_Target block) for each.  Because status and style are both part of a VCODE, there is no separate input for hand feedback status.  Note: any position information of these input VCODEs is overwritten by this block by the appropriate fingertip locations.
      | <P>
      | 
      | <H2>Related Blocks </H2>
      | DataLogging<BR>
      | Show_Target<BR>
      | Process_Video_CMD
      mask TypeOptions feedback_cntl_src: none | status only | style and status
  MATLAB Function : MATLAB Function  TreatAsAtomicUnit=on
      settings: PermitHierarchicalResolution=ParametersOnly
  hand feedback : Outport
  wires:
  template vcodes/1 -> Hand_Feedback/2(Contralateral_arm_VCODE), Hand_Feedback/1(Assess_arm_VCODE)
  Hand_Feedback/1(VCODE) -> MATLAB Function/1(feedback_vcodes)
  arm/1 -> MATLAB Function/2(arm_to_be_assessed)
  MATLAB Function/1(hand_vcodes) -> hand feedback/1

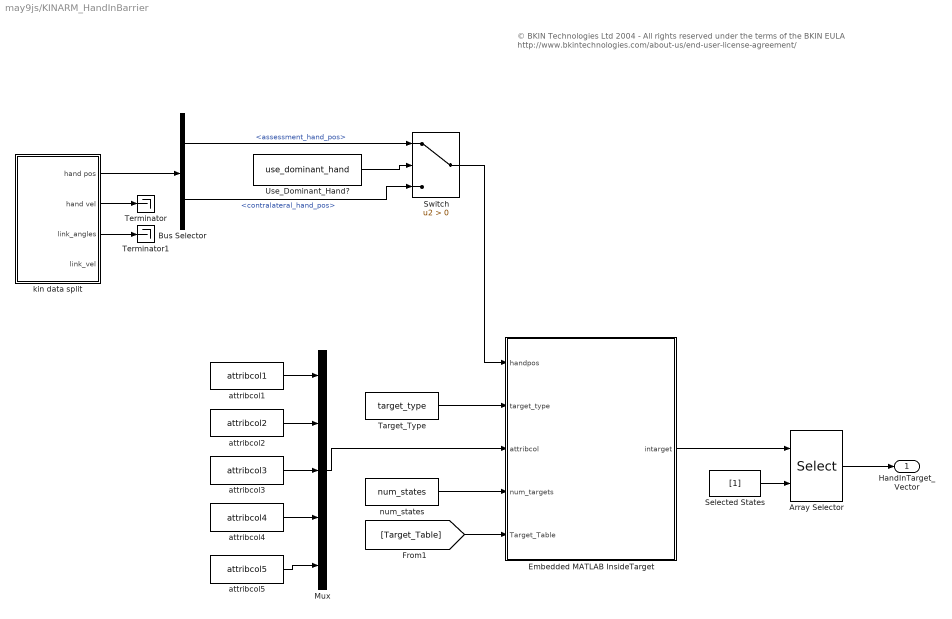
== system may9js/KINARM_HandInBarrier ==
  note: © BKIN Technologies Ltd 2004  - All rights reserved under the terms of the BKIN EULA
      | http://www.bkintechnologies.com/about-us/end-user-license-agreement/
  Array Selector : Selector  NumberOfDimensions=2  InputPortWidth=3  IndexOptions=Select all,Index vector (port)  Indices=-1,1  OutputSizes=slselsubs([(-2),(-2)],1),slselsubs([(-2),(-2)],2)
  Bus Selector : BusSelector  OutputSignals=assessment_hand_pos,contralateral_hand_pos
  Embedded MATLAB InsideTarget : MATLAB Function  TreatAsAtomicUnit=on
      settings: PermitHierarchicalResolution=ParametersOnly  RTWSystemCode=Nonreusable function  RTWFileNameOpts=Use function name
  Mux : Mux  Inputs=5
  Selected States : Constant  Value=[1]
  Switch : Switch  Criteria=u2 > Threshold
  Target_Type : Constant  Value=target_type
  Terminator : Terminator
  Terminator1 : Terminator
  Use_Dominant_Hand? : Constant  Value=use_dominant_hand
  attribcol1 : Constant  Value=attribcol1
  attribcol2 : Constant  Value=attribcol2
  attribcol3 : Constant  Value=attribcol3
  attribcol4 : Constant  Value=attribcol4
  attribcol5 : Constant  Value=attribcol5
  kin data split : Subsystem
  num_states : Constant  Value=num_states
  HandInTarget_Vector : Outport
  wires:
  Selected States/1 -> Array Selector/2
  num_states/1 -> Embedded MATLAB InsideTarget/4(num_targets)
  Mux/1 -> Embedded MATLAB InsideTarget/3(attribcol)
  attribcol4/1 -> Mux/4
  attribcol3/1 -> Mux/3
  attribcol2/1 -> Mux/2
  attribcol1/1 -> Mux/1
  Target_Type/1 -> Embedded MATLAB InsideTarget/2(target_type)
  Array Selector/1 -> HandInTarget_Vector/1
  [Target_Table] -> Embedded MATLAB InsideTarget/5(Target_Table)
  Embedded MATLAB InsideTarget/1(intarget) -> Array Selector/1
  attribcol5/1 -> Mux/5
  kin data split/1(hand pos) -> Bus Selector/1
  Use_Dominant_Hand?/1 -> Switch/2
  Bus Selector/1 -> Switch/1  "<assessment_hand_pos>"
  Bus Selector/2 -> Switch/3  "<contralateral_hand_pos>"
  kin data split/2(hand vel) -> Terminator/1
  kin data split/3(link_angles) -> Terminator1/1
  Switch/1 -> Embedded MATLAB InsideTarget/1(handpos)

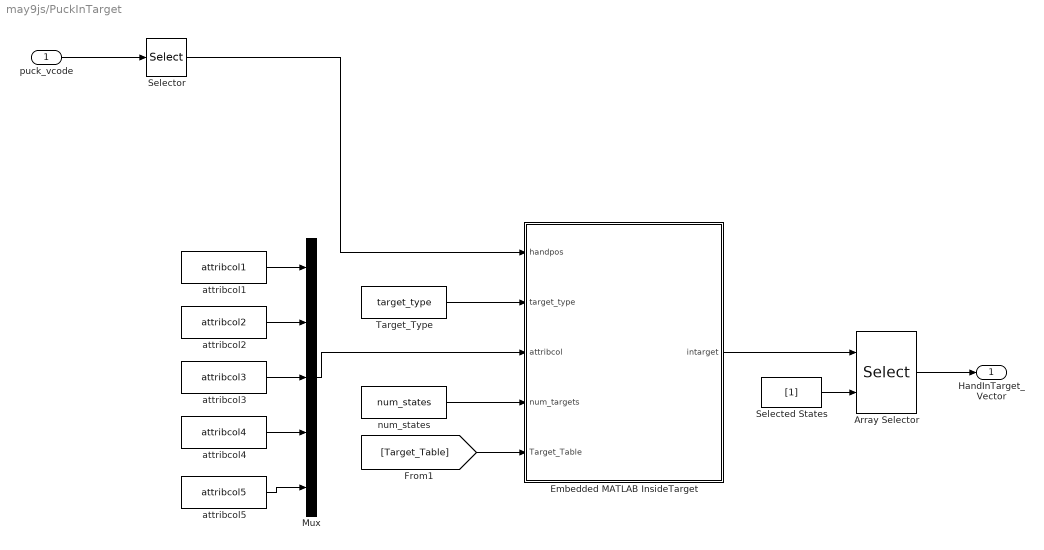
== system may9js/PuckInTarget ==
  puck_vcode : Inport  PortDimensions=[1,70]
  Array Selector : Selector  NumberOfDimensions=2  InputPortWidth=3  IndexOptions=Select all,Index vector (port)  Indices=-1,1  OutputSizes=slselsubs([(-2),(-2)],1),slselsubs([(-2),(-2)],2)
  Embedded MATLAB InsideTarget : MATLAB Function  TreatAsAtomicUnit=on
      settings: PermitHierarchicalResolution=ParametersOnly  RTWSystemCode=Nonreusable function  RTWFileNameOpts=Use function name
  Mux : Mux  Inputs=5
  Selected States : Constant  Value=[1]
  Selector : Selector  NumberOfDimensions=2  InputPortWidth=3  IndexOptions=Index vector (dialog),Index vector (dialog)  Indices=1,[3,4]  OutputSizes=1,1
  Target_Type : Constant  Value=target_type
  attribcol1 : Constant  Value=attribcol1
  attribcol2 : Constant  Value=attribcol2
  attribcol3 : Constant  Value=attribcol3
  attribcol4 : Constant  Value=attribcol4
  attribcol5 : Constant  Value=attribcol5
  num_states : Constant  Value=num_states
  HandInTarget_Vector : Outport
  wires:
  Selected States/1 -> Array Selector/2
  num_states/1 -> Embedded MATLAB InsideTarget/4(num_targets)
  Mux/1 -> Embedded MATLAB InsideTarget/3(attribcol)
  attribcol4/1 -> Mux/4
  attribcol3/1 -> Mux/3
  attribcol2/1 -> Mux/2
  attribcol1/1 -> Mux/1
  Target_Type/1 -> Embedded MATLAB InsideTarget/2(target_type)
  Array Selector/1 -> HandInTarget_Vector/1
  [Target_Table] -> Embedded MATLAB InsideTarget/5(Target_Table)
  Embedded MATLAB InsideTarget/1(intarget) -> Array Selector/1
  attribcol5/1 -> Mux/5
  Selector/1 -> Embedded MATLAB InsideTarget/1(handpos)
  puck_vcode/1 -> Selector/1
